simulink subsystem "rss_MotoSTMHybr"  (R2023a)
settings: Solver=VariableStepAuto  StartTime=0.0  StopTime=10.0  RelTol=1e-3
undefined symbols (not defined in the file): Cdbl_nElecAgSpdMaxVal, Cdbl_trqTqMaxVal, ENM_STRTUP_TRQ_STATUS, Gs16_nMinSenlRefElecSpd_C, Gs16_nOpnLpConvActElecSpd_C, Gs16_nShOffActElecSpd_C, Gs16_trqMinStrtUpRefTq_C, Gu16_phiMinOpnLpClsLpAgDvt_C
settings Model: Creator=xiaoqiang.yuan  LastModifiedBy=xiaoqiang.yuan

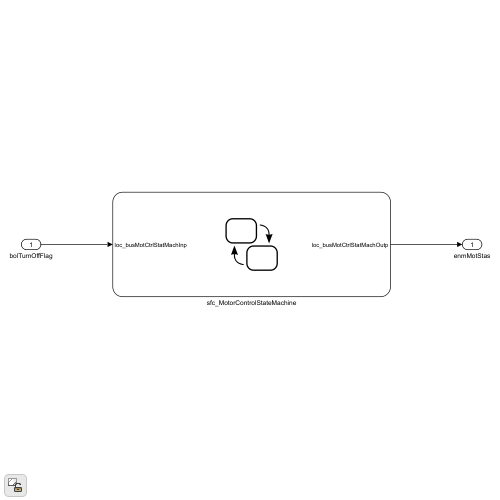
[thumbnail: Simulink's stored preview of the top-level diagram]
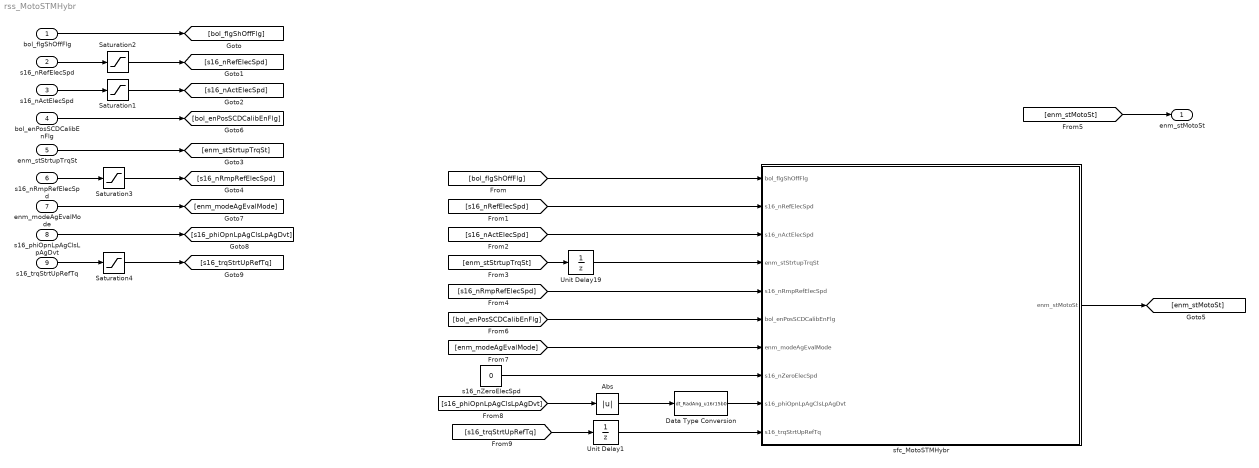
== system rss_MotoSTMHybr ==
  bol_flgShOffFlg : Inport  OutDataTypeStr=boolean
  s16_nRefElecSpd : Inport  Port=2  OutDataTypeStr=dt_Standardize_s16p15b0
  s16_nActElecSpd : Inport  Port=3  OutDataTypeStr=dt_Standardize_s16p15b0
  bol_enPosSCDCalibEnFlg : Inport  Port=4  OutDataTypeStr=boolean
  enm_stStrtupTrqSt : Inport  Port=5  OutDataTypeStr=Enum: ENM_STRTUP_TRQ_STATUS
  s16_nRmpRefElecSpd : Inport  Port=6  OutDataTypeStr=dt_Standardize_s16p15b0
  enm_modeAgEvalMode : Inport  Port=7  OutDataTypeStr=Enum: ENM_AG_POS_EVAL_MODE
  s16_phiOpnLpAgClsLpAgDvt : Inport  Port=8  OutDataTypeStr=dt_RadAng_s16r15b0
  s16_trqStrtUpRefTq : Inport  Port=9  OutDataTypeStr=dt_Standardize_s16p15b0
  Abs : Abs  SaturateOnIntegerOverflow=off
  Data Type Conversion : DataTypeConversion  OutDataTypeStr=dt_RadAng_u16r15b0  SaturateOnIntegerOverflow=off  RndMeth=Floor
  Saturation1 : Saturate  UpperLimit=Cdbl_nElecAgSpdMaxVal  LowerLimit=-Cdbl_nElecAgSpdMaxVal
  Saturation2 : Saturate  UpperLimit=Cdbl_nElecAgSpdMaxVal  LowerLimit=-Cdbl_nElecAgSpdMaxVal
  Saturation3 : Saturate  UpperLimit=Cdbl_nElecAgSpdMaxVal  LowerLimit=-Cdbl_nElecAgSpdMaxVal
  Saturation4 : Saturate  UpperLimit=Cdbl_trqTqMaxVal  LowerLimit=-Cdbl_trqTqMaxVal
  Unit Delay1 : UnitDelay  SampleTime=-1  HasFrameUpgradeWarning=on
  Unit Delay19 : UnitDelay  InitialCondition=ENM_STRTUP_TRQ_STATUS.TRQ_CST  SampleTime=-1  HasFrameUpgradeWarning=on
  s16_nZeroElecSpd : Constant  Value=0  OutDataTypeStr=dt_Standardize_s16p15b0
  sfc_MotoSTMHybr : Stateflow chart  TreatAsAtomicUnit=on
  enm_stMotoSt : Outport  OutDataTypeStr=Enum: ENM_MOTO_STATUS
  wires:
  enm_stStrtupTrqSt/1 -> [enm_stStrtupTrqSt]
  [enm_stStrtupTrqSt] -> Unit Delay19/1
  s16_nActElecSpd/1 -> Saturation1/1
  Saturation2/1 -> [s16_nRefElecSpd]
  [s16_nActElecSpd] -> sfc_MotoSTMHybr/3(s16_nActElecSpd)
  bol_flgShOffFlg/1 -> [bol_flgShOffFlg]
  [bol_flgShOffFlg] -> sfc_MotoSTMHybr/1(bol_flgShOffFlg)
  [enm_stMotoSt] -> enm_stMotoSt/1
  Unit Delay19/1 -> sfc_MotoSTMHybr/4(enm_stStrtupTrqSt)
  s16_nRmpRefElecSpd/1 -> Saturation3/1
  [s16_nRmpRefElecSpd] -> sfc_MotoSTMHybr/5(s16_nRmpRefElecSpd)
  s16_nRefElecSpd/1 -> Saturation2/1
  [s16_nRefElecSpd] -> sfc_MotoSTMHybr/2(s16_nRefElecSpd)
  Saturation1/1 -> [s16_nActElecSpd]
  sfc_MotoSTMHybr/1(enm_stMotoSt) -> [enm_stMotoSt]
  bol_enPosSCDCalibEnFlg/1 -> [bol_enPosSCDCalibEnFlg]
  enm_modeAgEvalMode/1 -> [enm_modeAgEvalMode]
  [bol_enPosSCDCalibEnFlg] -> sfc_MotoSTMHybr/6(bol_enPosSCDCalibEnFlg)
  [enm_modeAgEvalMode] -> sfc_MotoSTMHybr/7(enm_modeAgEvalMode)
  Saturation3/1 -> [s16_nRmpRefElecSpd]
  s16_nZeroElecSpd/1 -> sfc_MotoSTMHybr/8(s16_nZeroElecSpd)
  s16_phiOpnLpAgClsLpAgDvt/1 -> [s16_phiOpnLpAgClsLpAgDvt]
  [s16_phiOpnLpAgClsLpAgDvt] -> Abs/1
  s16_trqStrtUpRefTq/1 -> Saturation4/1
  [s16_trqStrtUpRefTq] -> Unit Delay1/1
  Saturation4/1 -> [s16_trqStrtUpRefTq]
  Unit Delay1/1 -> sfc_MotoSTMHybr/10(s16_trqStrtUpRefTq)
  Abs/1 -> Data Type Conversion/1
  Data Type Conversion/1 -> sfc_MotoSTMHybr/9(s16_phiOpnLpAgClsLpAgDvt)

== stateflow chart rss_MotoSTMHybr/sfc_MotoSTMHybr ==
  state OFF
    en:
    enm_stMotoSt = ENM_MOTO_STATUS.OFF;
  state OPEN_LOOP
    en:
    enm_stMotoSt = ENM_MOTO_STATUS.OPEN_LOOP;
  state CLOSED_LOOP
    en:
    enm_stMotoSt = ENM_MOTO_STATUS.CLOSED_LOOP;
  (default) -> OFF
  (junction 14) -> OFF
  CLOSED_LOOP -> (junction 14) [order 1] : [(s16_nRefElecSpd == s16_nZeroElecSpd && ...
      | abs(s16_nActElecSpd) < abs(Gs16_nShOffActElecSpd_C) &&...
      | not(bol_enPosSCDCalibEnFlg)) || ...
      | bol_flgShOffFlg]
  OFF -> (junction 124) : [(abs(s16_nRefElecSpd) > s16_nZeroElecSpd || ...
      | bol_enPosSCDCalibEnFlg ) && ...
      | not(bol_flgShOffFlg)]
  (junction 124) -> (junction 6)
  OPEN_LOOP -> OFF [order 2] : [(s16_nRefElecSpd == s16_nZeroElecSpd && ...
      | abs(s16_nActElecSpd) < abs(Gs16_nShOffActElecSpd_C) &&...
      | not(bol_enPosSCDCalibEnFlg)) || ...
      | bol_flgShOffFlg]
  (junction 6) -> OPEN_LOOP [order 2]
  (junction 6) -> CLOSED_LOOP [order 1] : [enm_modeAgEvalMode ~= ENM_AG_POS_EVAL_MODE.SENSORLESS]
  OPEN_LOOP -> CLOSED_LOOP [order 1] : [enm_stStrtupTrqSt == ENM_STRTUP_TRQ_STATUS.TRQ_DECRE &&...
      | (s16_phiOpnLpAgClsLpAgDvt <= Gu16_phiMinOpnLpClsLpAgDvt_C || abs(s16_trqStrtUpRefTq) <= abs(Gs16_trqMinStrtUpRefTq_C))]
  CLOSED_LOOP -> OPEN_LOOP [order 2] : [s16_nRefElecSpd ~= s16_nZeroElecSpd && abs(s16_nRmpRefElecSpd) < abs(Gs16_nMinSenlRefElecSpd_C) &&...
      |  abs(s16_nActElecSpd) < abs(Gs16_nOpnLpConvActElecSpd_C) && ...
      | enm_modeAgEvalMode == ENM_AG_POS_EVAL_MODE.SENSORLESS]
  data: Gs16_nShOffActElecSpd_C parameter; Gs16_nMinSenlRefElecSpd_C parameter; Gs16_nOpnLpConvActElecSpd_C parameter; bol_flgShOffFlg input boolean; s16_nRefElecSpd input dt_Standardize_s16p15b0; s16_nActElecSpd input dt_Standardize_s16p15b0; enm_stMotoSt output Enum: ENM_MOTO_STATUS; enm_stStrtupTrqSt input Enum: ENM_STRTUP_TRQ_STATUS; s16_nRmpRefElecSpd input dt_Standardize_s16p15b0; bol_enPosSCDCalibEnFlg input boolean; enm_modeAgEvalMode input Enum: ENM_AG_POS_EVAL_MODE; s16_nZeroElecSpd input dt_Standardize_s16p15b0; s16_phiOpnLpAgClsLpAgDvt input dt_RadAng_u16r15b0; s16_trqStrtUpRefTq input dt_Standardize_s16p15b0; Gu16_phiMinOpnLpClsLpAgDvt_C parameter; Gs16_trqMinStrtUpRefTq_C parameter
